simulink model "FIR_TDM_Ex_1"  (R2023b)
settings: Solver=VariableStepAuto  StartTime=0.0  StopTime=10  RelTol=1e-3
undefined symbols (not defined in the file): Asymmetric, coeffs, S, vsva2197, xcvc1902
libraries: aieDSP x1, vmcUtilities x1
settings Model: Creator=sdegala  LastModifiedBy=sdegala

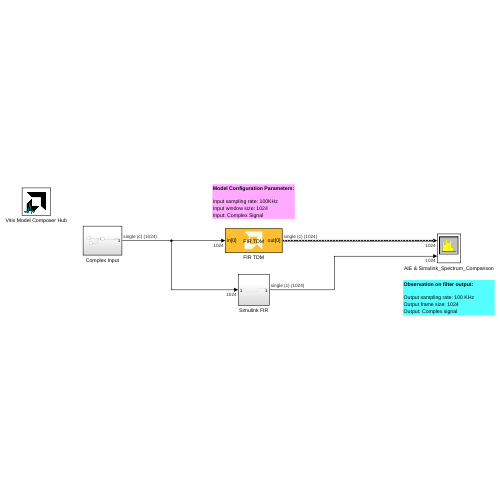
[thumbnail: Simulink's stored preview of the top-level diagram]
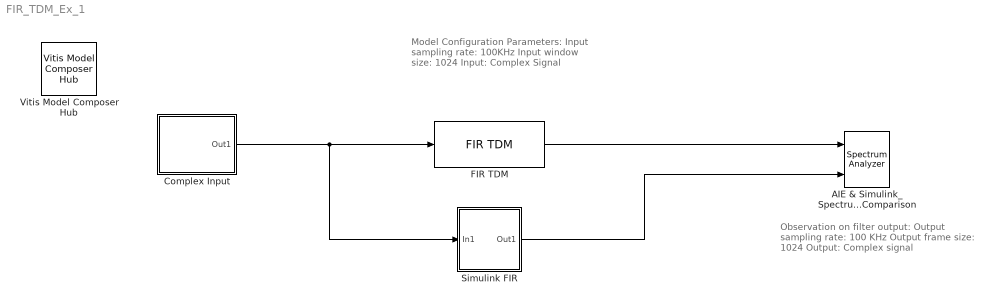
== system FIR_TDM_Ex_1 ==
  note: Observation on filter output:
      |
      | Output sampling rate: 100 KHz
      | Output frame size: 1024
      | Output: Complex signal
  note: Model Configuration Parameters:
      |
      | Input sampling rate: 100KHz
      | Input window size: 1024
      | Input: Complex Signal
  AIE & Simulink_Spectrum_Comparison : SpectrumAnalyzer  NumInputPorts=2  WindowPosition=[1.000000,37.000000,1280.000000,735.000000,]  Visible=on  ScopeFrameLocation=window  SampleRate=100000  Span=99999.99999999999  StartFrequency=-49999.99999999999  StopFrequency=49999.99999999999  AveragingMethod=Exponential  YLimits=[-207.77909733,102.43132807]  ShowLegend=on  SelectedToolstripTab=spectrumAnalyzerToolstrip.spectrumTab  DefaultConfigurationName=spbscopes.SpectrumAnalyzerBlockCfg  IsFrequencyInputMode=0  FrequencyVectorPort=0  FrequencyVectorFromPort=0  FrequencyInputRBWPort=0  FrequencyInputRBWFromPort=0
  Complex Input : Subsystem
  FIR TDM : aieDSP/FIR TDM  data_type=cfloat  coef_type=float  num_outputs=off  dual_ip=off  fir_length=16  coeff=coeffs_AIE  shift_val=0  rnd_mode=Floor  input_window_size=1024  tdm_channels=8  sat_mode=1-Asymmetric  AIE_VARIANT=1  blockJsonConstraints=[]  blockJsonConstraintsInternal=[]  spec=vmc_fir_tdm.json  SerializedMaskParamNames=[]  SerializedMaskParamValues=[]  SerializedMaskParamVisibilities=[]  block_type=FIR TDM  SerializedMaskParamDataypes=typename|typename|bool|bool|uint|coef_type|uint|uint|uint|uint|uint|uint  SerializedMaskParamEnumStrArr=0|0|0|0|0|0|0|Floor,Ceiling,Round to positive infinity,Round to negative infinity,Round symmetrical to infinity,Round symmetrical to zero,Round convergent to even,Round convergent to odd|0|0|0-None,1-Asymmetric,3-Symmetric|0  SerializedMaskParamEnumValArr=0|0|0|0|0|0|0|0,1,2,3,4,5,6,7|0|0|0,1,3|0  SerializedMaskParamVectorArr=0|0|0|0|0|1|0|0|0|0|0|0
  Simulink FIR : Subsystem
  Vitis Model Composer Hub : vmcUtilities/Vitis Model Composer Hub  Tag=genX  CodeGeneration=off  TargetDirectory=./code  exportDesign=off  analyzeDesign=off  validateDesignOnHw=off  ExportType=AI Engines  IpVendor=xilinx.com  IpLibrary=hls  IpVersion=1.0  IpHWLanguage=Verilog  AieCompilerOptions={}  AieSimulatorOptions={}  CreateTestbench=off  TestbenchStackSize=10  RunRtlSim=off  RunCSim=off  RunAieSim=off  AieSimTimeout=50000  RunAieSimProfiling=off  LaunchVitisAnalyzer=off  PlotOutput=off  RunX86Sim=off  X86SimTimeout=10  GenHwImage=off  GenLibadfXo=off  GenHwValidationCode=off  PlatformType=Not Specified  HwSystemType=Baremetal  HwValidationTarget=hw  ProjDevice=xcvc1902-vsva2197-1LP-e-S  ProjDevicePart=xcvc1902-vsva2197-1LP-e-S  AIEType=AIE  SamplePeriod=-1  ClockFrequency=200  DataPathParallelism=1  xilinxfamily=versalaicore  part=xcvc1902  speed=-1LP-e-S  package=vsva2197  directory=./netlist  testbench=off  incr_netlist=off  synthesis_tool=Vivado  clock_wrapper=Clock Enables  dbl_ovrd=According to Block Masks  dcm_input_clock_period=10  sysclk_period=10  simulink_period=1  eval_field=0  LogFileName=''  NThreads=4
  wires:
  FIR TDM/1 -> AIE & Simulink_Spectrum_Comparison/1
  Complex Input/1(Out1) -> Simulink FIR/1(In1), FIR TDM/1
  Simulink FIR/1(Out1) -> AIE & Simulink_Spectrum_Comparison/2

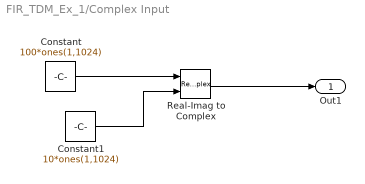
== system FIR_TDM_Ex_1/Complex Input ==
  Constant : Constant  Value=100*ones(1,1024)  OutDataTypeStr=single  SampleTime=1/100e3
  Constant1 : Constant  Value=10*ones(1,1024)  OutDataTypeStr=single  SampleTime=1/100e3
  Real-Imag to Complex : RealImagToComplex
  Out1 : Outport
  wires:
  Constant/1 -> Real-Imag to Complex/1
  Constant1/1 -> Real-Imag to Complex/2
  Real-Imag to Complex/1 -> Out1/1

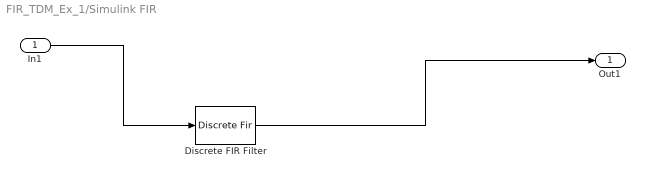
== system FIR_TDM_Ex_1/Simulink FIR ==
  In1 : Inport
  Discrete FIR Filter : DiscreteFir  Coefficients=coeffs  InputProcessing=Columns as channels (frame based)  RndMeth=Round
  Out1 : Outport
  wires:
  In1/1 -> Discrete FIR Filter/1
  Discrete FIR Filter/1 -> Out1/1
